simulink model "CSE_STEPRESPONSE_BLOCKDIAGRAM_NO8_FAJANILAN"  (R2019a)
settings: Solver=VariableStepAuto  StartTime=0.0  StopTime=20  RelTol=1e-3
values from neighbouring files (symbols this model uses):
  G_den8 = [1 3 5 7 9 1]    [CSE_STEPRESPONSE_CODE_NO7_NO8_FAJANILAN.m]    (also in CSE_STEPRESPONSE_CODE_NO8_FAJANILAN.m)
  G_num8 = [10 8 6 4 2]    [CSE_STEPRESPONSE_CODE_NO7_NO8_FAJANILAN.m]    (also in CSE_STEPRESPONSE_CODE_NO8_FAJANILAN.m)
settings Model: Creator=Liza Encarnado  LastModifiedBy=Liza Encarnado

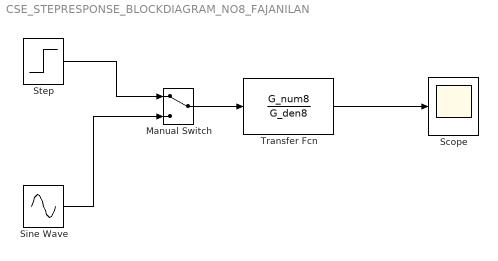
== system CSE_STEPRESPONSE_BLOCKDIAGRAM_NO8_FAJANILAN ==
  Manual Switch : ManualSwitch
  Scope : Scope
  Sine Wave : Sin  SampleTime=0
  Step : Step  Time=0  SampleTime=0
  Transfer Fcn : TransferFcn  Numerator=G_num8  Denominator=G_den8
  wires:
  Step/1 -> Manual Switch/1
  Transfer Fcn/1 -> Scope/1
  Sine Wave/1 -> Manual Switch/2
  Manual Switch/1 -> Transfer Fcn/1
